simulink model "generic_20231123_1032"  (R2022b)
settings: Solver=ode45  StartTime=0.0  StopTime=50  RelTol=1e-3  EnableMultiTasking=on
model workspace (MAT data in the model file):
  A = 1
  Amplifier = -9.10007585438
  B = 1.19071237887
  K_d_yawrate = 0.231634180251
  K_dsteering = 5.24463953925
  k_speed = -0.570636497542
  k_stanley = 28.4909595466
  kd = -9.99955278144
  ki = 0.00519416981022
  kp = 9.99999979837
  path_curvature = 0
values from neighbouring files (symbols this model uses):
  brake_select = ones(length(speed), length(steering_angle))    [TwoDLook_uptable.m]
  curvature = 0.000:0.001:1    [TwoDLook_uptable.m]
  m = 1600    [MPCController1.m]    (also in MPCController2.m; MPC_Fmincon.m)
  speed = 0:0.1:100    [TwoDLook_uptable.m]
  steering_angle = -3.14/4:0.00628/4:3.14/4    [TwoDLook_uptable.m]
undefined symbols (not defined in the file or in its folder): DiscIntNeverNeededParam
libraries: CarMaker4SL x143, simulink x11, cstblocks x6, simulink_extras x4, autolibshared x1, mpcadaslib x1
(part 4 of 7)

== system generic_20231123_1032/CarMaker/VehicleControl/CreateBus VhclCtrl/Stanley steering & speed//Brake controller/Road sensor set & path planning/Road sensor set & path planning/Be'zeir path planning ==
  pathx : Inport
  path_y : Inport  Port=2
  car_v : Inport  Port=3
  Basic_obstacle avoidance : MATLAB Function  TreatAsAtomicUnit=on
  Constant : Constant  Value=10
  Constant1 : Constant  Value=1.95
  Constant2 : Constant  Value=4.2
  Demux : Demux
  Discrete-Time Integrator : DiscreteIntegrator  SampleTime=-1  ICPrevOutput=DiscIntNeverNeededParam  ICPrevScaledInput=DiscIntNeverNeededParam
  MATLAB Function : MATLAB Function  TreatAsAtomicUnit=on
  Mux : Mux  Inputs=2
  Mux1 : Mux  Inputs=2
  Read CM Dict : CarMaker4SL/Read CM Dict  xname=Sensor.Object.RadarL.Obj.T00.RefPnt.ds.x  xsync=off  xstime=Continuous
  Read CM Dict1 : CarMaker4SL/Read CM Dict  xname=Sensor.Object.RadarL.Obj.T00.RefPnt.ds.y  xsync=off  xstime=Continuous
  Read CM Dict2 : CarMaker4SL/Read CM Dict  xname=Car.Gen.tx  xsync=off  xstime=Continuous
  Read CM Dict3 : CarMaker4SL/Read CM Dict  xname=Car.Gen.ty  xsync=off  xstime=Continuous
  Read CM Dict4 : CarMaker4SL/Read CM Dict  xname=Sensor.Radar.VehSensor_6.Obj0.Width  xsync=off  xstime=Continuous
  Read CM Dict5 : CarMaker4SL/Read CM Dict  xname=Sensor.Radar.VehSensor_6.Obj0.Length  xsync=off  xstime=Continuous
  Read CM Dict6 : CarMaker4SL/Read CM Dict  xname=Car.YawRate  xsync=off  xstime=Continuous
  Reshape : Reshape  OutputDimensionality=Customize  OutputDimensions=[2,1]
  Reshape1 : Reshape  OutputDimensionality=Customize  OutputDimensions=[1,2]
  Reshape2 : Reshape  OutputDimensionality=Customize  OutputDimensions=[1,2]
  Reshape3 : Reshape  OutputDimensionality=Customize  OutputDimensions=[1,2]
  Reshape4 : Reshape
  Saturation : Saturate  UpperLimit=4  LowerLimit=-4
  Signal_smoothing : Subsystem
  Smoothing3 : Subsystem
  getInstantaneousPath Function : MATLAB Function  Commented=on  TreatAsAtomicUnit=on
  lookahead_dist : Constant  Commented=on  Value=2
  new_x_path : Outport
  new_y_path : Outport  Port=2
  wires:
  Read CM Dict1/1 -> Basic_obstacle avoidance/8(dy), MATLAB Function/4(dx)
  Read CM Dict2/1 -> Mux/1
  MATLAB Function/2(final_position) -> Reshape3/1
  Constant/1 -> MATLAB Function/5(path_length)
  Read CM Dict4/1 -> Signal_smoothing/1(Signal_In)
  Read CM Dict3/1 -> Mux/2
  Mux/1 -> Reshape/1
  Read CM Dict6/1 -> Discrete-Time Integrator/1
  Read CM Dict5/1 -> Saturation/1
  Mux1/1 -> Reshape1/1
  Read CM Dict/1 -> Basic_obstacle avoidance/7(dx), MATLAB Function/3(dy)
  Reshape/1 -> getInstantaneousPath Function/3(current_position), MATLAB Function/1(current_position)
  Discrete-Time Integrator/1 -> MATLAB Function/2(heading), getInstantaneousPath Function/4(current_heading)
  Saturation/1 -> Smoothing3/1(Signal_In)
  MATLAB Function/1(initial_position) -> Reshape2/1
  Signal_smoothing/1(smoothed_width) -> Basic_obstacle avoidance/3(obstacle_width)
  Constant1/1 -> Basic_obstacle avoidance/5(car_width)
  Smoothing3/1(Signal_Out) -> Basic_obstacle avoidance/4(obstacle_length)  "steering_signal"
  Constant2/1 -> Basic_obstacle avoidance/6(car_length)
  car_v/1 -> Basic_obstacle avoidance/9(car_v)
  path_y/1 -> Mux1/2, Basic_obstacle avoidance/11(path_y)
  pathx/1 -> Mux1/1, Basic_obstacle avoidance/10(path_x)
  lookahead_dist/1 -> getInstantaneousPath Function/2(lookahead_distance)
  Reshape2/1 -> Basic_obstacle avoidance/1(initial_position)
  Reshape3/1 -> Basic_obstacle avoidance/2(final_position)
  Demux/1 -> new_x_path/1
  Basic_obstacle avoidance/1(updated_path) -> Reshape4/1, getInstantaneousPath Function/1(generated_path)
  Demux/4 -> new_y_path/1
  Reshape4/1 -> Demux/1

== system generic_20231123_1032/CarMaker/VehicleControl/CreateBus VhclCtrl/Stanley steering & speed//Brake controller/Road sensor set & path planning/Road sensor set & path planning/Car_yaw_rate ==
  Velocity : Inport
  X-path : Inport  Port=2
  Y_path : Inport  Port=3
  " Path_expanding1" : Subsystem
  Constant : Constant  Value=20
  Gain2 : Gain  Gain=-1
  Multiport Switch : MultiPortSwitch  Inputs=2  SaturateOnIntegerOverflow=off  InputSameDT=off
  Multiport Switch1 : MultiPortSwitch  Inputs=2  SaturateOnIntegerOverflow=off  InputSameDT=off
  Product3 : Product
  Read CM Dict5 : CarMaker4SL/Read CM Dict  xname=Car.YawRate  xsync=off  xstime=Continuous
  Saturation3 : Saturate  UpperLimit=5  LowerLimit=-5
  Varying Lowpass Filter1 : cstblocks/Linear Parameter Varying/Varying Lowpass Filter  N=1
  Vehicle_yaw_rate_selcotr : Constant
  Yaw_rate_filter_slector : Constant
  calculate_path_curvature2 : MATLAB Function  TreatAsAtomicUnit=on  VariantControl=Choice
  Yaw_rate_car : Outport
  wires:
  " Path_expanding1"/1(x_path) -> calculate_path_curvature2/1(path_x)
  X-path/1 -> " Path_expanding1"/1(X-path)
  Gain2/1 -> Multiport Switch1/2, Saturation3/1
  Y_path/1 -> " Path_expanding1"/2(Y_path)
  Velocity/1 -> Product3/1
  " Path_expanding1"/2(y_path) -> calculate_path_curvature2/2(path_y)
  Product3/1 -> Gain2/1
  calculate_path_curvature2/1(path_curvature) -> Product3/2
  Saturation3/1 -> Varying Lowpass Filter1/1
  Constant/1 -> Varying Lowpass Filter1/2
  Yaw_rate_filter_slector/1 -> Multiport Switch1/1
  Varying Lowpass Filter1/1 -> Multiport Switch1/3  "Yaw_rate_car"
  Vehicle_yaw_rate_selcotr/1 -> Multiport Switch/1
  Multiport Switch1/1 -> Multiport Switch/2
  Read CM Dict5/1 -> Multiport Switch/3
  Multiport Switch/1 -> Yaw_rate_car/1  "Yaw_rate_car"

== system generic_20231123_1032/CarMaker/VehicleControl/CreateBus VhclCtrl/Stanley steering & speed//Brake controller/Road sensor set & path planning/Road sensor set & path planning/Cross_track_error_calcuation ==
  x_path : Inport
  y_path : Inport  Port=2
  Constant : Constant  Value=25
  Cross_track_error_calcuation : MATLAB Function  TreatAsAtomicUnit=on
  Delay : Delay  DelayLength=1  InitialCondition=0.1
  Delay1 : Delay  DelayLength=1  InitialCondition=0.1
  Gain1 : Gain  Gain=-1
  Read CM Dict12 : CarMaker4SL/Read CM Dict  xname=Car.Gen.ty  xsync=off  xstime=Continuous
  Read CM Dict8 : CarMaker4SL/Read CM Dict  xname=Car.Gen.tx  xsync=off  xstime=Continuous
  Saturation1 : Saturate  UpperLimit=7  LowerLimit=-7
  Varying Lowpass Filter2 : cstblocks/Linear Parameter Varying/Varying Lowpass Filter  N=1
  cte : Outport
  denominator : Outport  Port=2
  wires:
  Read CM Dict12/1 -> Cross_track_error_calcuation/2(y_vehicle)
  x_path/1 -> Cross_track_error_calcuation/5(x2), Delay1/1
  Saturation1/1 -> Varying Lowpass Filter2/1
  Delay/1 -> Cross_track_error_calcuation/4(y_point)
  Cross_track_error_calcuation/2(denominator) -> denominator/1
  y_path/1 -> Cross_track_error_calcuation/6(y2), Delay/1
  Delay1/1 -> Cross_track_error_calcuation/3(x_point)
  Read CM Dict8/1 -> Cross_track_error_calcuation/1(x_vehicle)
  Cross_track_error_calcuation/1(cte) -> Gain1/1
  Gain1/1 -> Saturation1/1
  Constant/1 -> Varying Lowpass Filter2/2
  Varying Lowpass Filter2/1 -> cte/1

== system generic_20231123_1032/CarMaker/VehicleControl/CreateBus VhclCtrl/Stanley steering & speed//Brake controller/Road sensor set & path planning/Road sensor set & path planning/Dijkestra path planning ==
  path_y : Inport
  car_v : Inport  Port=2
  pathx : Inport  Port=3
  Basic_obstacle avoidance : MATLAB Function  TreatAsAtomicUnit=on
  Demux : Demux  Commented=on
  Discrete-Time Integrator : DiscreteIntegrator  SampleTime=-1  ICPrevOutput=DiscIntNeverNeededParam  ICPrevScaledInput=DiscIntNeverNeededParam
  Mux : Mux  Inputs=2
  Mux1 : Mux  Inputs=2
  Read CM Dict : CarMaker4SL/Read CM Dict  xname=Sensor.Object.RadarL.Obj.T00.RefPnt.ds.x  xsync=off  xstime=Continuous
  Read CM Dict1 : CarMaker4SL/Read CM Dict  xname=Sensor.Object.RadarL.Obj.T00.RefPnt.ds.y  xsync=off  xstime=Continuous
  Read CM Dict2 : CarMaker4SL/Read CM Dict  xname=Car.Gen.tx  xsync=off  xstime=Continuous
  Read CM Dict3 : CarMaker4SL/Read CM Dict  xname=Car.Gen.ty  xsync=off  xstime=Continuous
  Read CM Dict4 : CarMaker4SL/Read CM Dict  xname=Sensor.Radar.VehSensor_6.Obj0.Width  xsync=off  xstime=Continuous
  Read CM Dict5 : CarMaker4SL/Read CM Dict  xname=Sensor.Radar.VehSensor_6.Obj0.Length  xsync=off  xstime=Continuous
  Read CM Dict6 : CarMaker4SL/Read CM Dict  xname=Car.YawRate  xsync=off  xstime=Continuous
  Reshape : Reshape  OutputDimensionality=Customize  OutputDimensions=[2,1]
  Reshape1 : Reshape  OutputDimensionality=Customize  OutputDimensions=[1,2]
  Reshape4 : Reshape  Commented=on
  Saturation : Saturate  UpperLimit=4  LowerLimit=-4
  Signal_smoothing : Subsystem
  Smoothing3 : Subsystem
  getInstantaneousPath Function : MATLAB Function  Commented=on  TreatAsAtomicUnit=on
  lookahead_dist : Constant  Commented=on  Value=2
  new_x_path : Outport
  new_y_path : Outport  Port=2
  wires:
  Read CM Dict/1 -> Basic_obstacle avoidance/3(dx)
  Read CM Dict1/1 -> Basic_obstacle avoidance/4(dy)
  Read CM Dict2/1 -> Mux/1, Basic_obstacle avoidance/1(Car_x)
  Read CM Dict4/1 -> Signal_smoothing/1(Signal_In)
  Read CM Dict3/1 -> Mux/2, Basic_obstacle avoidance/2(Car_y)
  Mux/1 -> Reshape/1
  Read CM Dict6/1 -> Discrete-Time Integrator/1
  Read CM Dict5/1 -> Saturation/1
  Mux1/1 -> Reshape1/1
  Reshape/1 -> getInstantaneousPath Function/3(current_position)
  Discrete-Time Integrator/1 -> getInstantaneousPath Function/4(current_heading)
  Saturation/1 -> Smoothing3/1(Signal_In)
  Signal_smoothing/1(smoothed_width) -> Basic_obstacle avoidance/6(object_width)
  Smoothing3/1(Signal_Out) -> Basic_obstacle avoidance/5(object_length)  "steering_signal"
  car_v/1 -> Basic_obstacle avoidance/7(car_v)
  path_y/1 -> Mux1/2, Basic_obstacle avoidance/9(path_y)
  pathx/1 -> Mux1/1, Basic_obstacle avoidance/8(path_x)
  lookahead_dist/1 -> getInstantaneousPath Function/2(lookahead_distance)
  Demux/1 -> new_x_path/1
  Basic_obstacle avoidance/1(updated_path) -> Reshape4/1, getInstantaneousPath Function/1(generated_path)
  Demux/4 -> new_y_path/1
  Reshape4/1 -> Demux/1

== system generic_20231123_1032/CarMaker/VehicleControl/CreateBus VhclCtrl/Stanley steering & speed//Brake controller/Road sensor set & path planning/Road sensor set & path planning/Path_curvature ==
  X-path : Inport
  Y_path : Inport  Port=2
  " Path_expanding" : Subsystem
  Constant : Constant  Value=25
  Multiport Switch : MultiPortSwitch  Inputs=2  SaturateOnIntegerOverflow=off  InputSameDT=off
  Multiport Switch1 : MultiPortSwitch  Inputs=2  SaturateOnIntegerOverflow=off  InputSameDT=off
  Read CM Dict6 : CarMaker4SL/Read CM Dict  xname=Sensor.Road.VehSensor_0.Path.CurveXY  xsync=off  xstime=Continuous
  Saturation2 : Saturate  UpperLimit=1  LowerLimit=-1
  Scope : Scope
  Varying Lowpass Filter : cstblocks/Linear Parameter Varying/Varying Lowpass Filter  N=1
  calculate_path_curvature1 : MATLAB Function  TreatAsAtomicUnit=on  VariantControl=Choice
  inverting : Gain  Gain=-1
  path_curv_selector : Constant
  path_curv_selector1 : Constant
  Path_curvature : Outport
  smoothed_path_curvature : Outport  Port=2
  wires:
  inverting/1 -> Multiport Switch1/2, Saturation2/1
  X-path/1 -> " Path_expanding"/1(X-path)
  Y_path/1 -> " Path_expanding"/2(Y_path)
  " Path_expanding"/1(x_path) -> calculate_path_curvature1/1(path_x)
  calculate_path_curvature1/1(path_curvature) -> inverting/1
  Read CM Dict6/1 -> Multiport Switch/3
  " Path_expanding"/2(y_path) -> calculate_path_curvature1/2(path_y)
  Saturation2/1 -> Varying Lowpass Filter/1
  Varying Lowpass Filter/1 -> Scope/1, smoothed_path_curvature/1, Multiport Switch1/3  "Path_curvature"
  Constant/1 -> Varying Lowpass Filter/2
  path_curv_selector1/1 -> Multiport Switch1/1
  path_curv_selector/1 -> Multiport Switch/1
  Multiport Switch1/1 -> Multiport Switch/2
  Multiport Switch/1 -> Path_curvature/1  "Path_curvature"

== system generic_20231123_1032/CarMaker/VehicleControl/CreateBus VhclCtrl/Stanley steering & speed//Brake controller/Road sensor set & path planning/Road sensor set & path planning/Spline_path_planning ==
  Velocity : Inport
  pathx : Inport  Port=2
  path_y : Inport  Port=3
  Demux : Demux  Outputs=2
  Discrete-Time Integrator : DiscreteIntegrator  SampleTime=-1  ICPrevOutput=DiscIntNeverNeededParam  ICPrevScaledInput=DiscIntNeverNeededParam
  Mux : Mux  Inputs=2
  Mux1 : Mux  Inputs=2
  Read CM Dict : CarMaker4SL/Read CM Dict  xname=Sensor.Object.RadarL.Obj.T00.RefPnt.ds.x  xsync=off  xstime=Continuous
  Read CM Dict1 : CarMaker4SL/Read CM Dict  xname=Sensor.Object.RadarL.Obj.T00.RefPnt.ds.y  xsync=off  xstime=Continuous
  Read CM Dict2 : CarMaker4SL/Read CM Dict  xname=Car.Gen.tx  xsync=off  xstime=Continuous
  Read CM Dict3 : CarMaker4SL/Read CM Dict  xname=Car.Gen.ty  xsync=off  xstime=Continuous
  Read CM Dict4 : CarMaker4SL/Read CM Dict  xname=Sensor.Radar.VehSensor_6.Obj0.Width  xsync=off  xstime=Continuous
  Read CM Dict5 : CarMaker4SL/Read CM Dict  xname=Sensor.Radar.VehSensor_6.Obj0.Length  xsync=off  xstime=Continuous
  Read CM Dict6 : CarMaker4SL/Read CM Dict  xname=Car.YawRate  xsync=off  xstime=Continuous
  Reshape : Reshape  OutputDimensionality=Customize  OutputDimensions=[1,2]
  Reshape1 : Reshape  OutputDimensionality=Customize  OutputDimensions=[1,2]
  Saturation : Saturate  UpperLimit=4  LowerLimit=-4
  Signal_smoothing : Subsystem
  Smoothing3 : Subsystem
  Spline_bsed_obstacle avoidance : MATLAB Function  TreatAsAtomicUnit=on
  getInstantaneousPath Function : MATLAB Function  TreatAsAtomicUnit=on
  lookahead_dist : Constant  Value=2
  new_x_path : Outport
  new_y_path : Outport  Port=2
  wires:
  Signal_smoothing/1(smoothed_width) -> Spline_bsed_obstacle avoidance/5(object_width)
  Read CM Dict4/1 -> Signal_smoothing/1(Signal_In)
  Demux/1 -> new_x_path/1
  Demux/2 -> new_y_path/1
  Spline_bsed_obstacle avoidance/1(updated_path) -> getInstantaneousPath Function/1(generated_path)  "generated_path"
  Smoothing3/1(Signal_Out) -> Spline_bsed_obstacle avoidance/6(object_length)  "steering_signal"
  Read CM Dict1/1 -> Spline_bsed_obstacle avoidance/4(dy)
  Read CM Dict/1 -> Spline_bsed_obstacle avoidance/3(dx)
  Saturation/1 -> Smoothing3/1(Signal_In)
  Velocity/1 -> Spline_bsed_obstacle avoidance/7(car_v)
  Read CM Dict5/1 -> Saturation/1
  Read CM Dict3/1 -> Mux/2, Spline_bsed_obstacle avoidance/2(Car_y)  "car_y"
  Read CM Dict2/1 -> Mux/1, Spline_bsed_obstacle avoidance/1(Car_x)  "car_x"
  Mux/1 -> Reshape/1
  Reshape/1 -> getInstantaneousPath Function/3(current_position)
  lookahead_dist/1 -> getInstantaneousPath Function/2(lookahead_distance)
  Read CM Dict6/1 -> Discrete-Time Integrator/1
  Discrete-Time Integrator/1 -> getInstantaneousPath Function/4(current_heading)
  Mux1/1 -> Reshape1/1
  pathx/1 -> Spline_bsed_obstacle avoidance/8(pathx), Mux1/1
  path_y/1 -> Spline_bsed_obstacle avoidance/9(path_y), Mux1/2
  getInstantaneousPath Function/1(instantaneous_points) -> Demux/1

== system generic_20231123_1032/CarMaker/VehicleControl/CreateBus VhclCtrl/Stanley steering & speed//Brake controller/Road sensor set & path planning/Road sensor set & path planning/path_planning ==
  <tx> : Inport
  <ty> : Inport  Port=2
  Velocity : Inport  Port=3
  Basic_obstacle avoidance : MATLAB Function  TreatAsAtomicUnit=on
  Demux : Demux  Outputs=2
  Floor : Rounding  Operator=ceil
  Read CM Dict : CarMaker4SL/Read CM Dict  xname=Sensor.Object.RadarL.Obj.T00.RefPnt.ds.x  xsync=off  xstime=Continuous
  Read CM Dict1 : CarMaker4SL/Read CM Dict  xname=Sensor.Object.RadarL.Obj.T00.RefPnt.ds.y  xsync=off  xstime=Continuous
  Read CM Dict2 : CarMaker4SL/Read CM Dict  xname=Car.Gen.tx  xsync=off  xstime=Continuous
  Read CM Dict3 : CarMaker4SL/Read CM Dict  xname=Car.Gen.ty  xsync=off  xstime=Continuous
  Read CM Dict4 : CarMaker4SL/Read CM Dict  xname=Sensor.Radar.VehSensor_6.Obj0.Width  xsync=off  xstime=Continuous
  Read CM Dict5 : CarMaker4SL/Read CM Dict  xname=Sensor.Radar.VehSensor_6.Obj0.Length  xsync=off  xstime=Continuous
  Saturation : Saturate  UpperLimit=4  LowerLimit=-4
  Signal_smoothing : Subsystem
  Smoothing3 : Subsystem
  To Workspace1 : ToWorkspace  Commented=on  VariableName=CarY  SampleTime=-1
      settings: Save2DSignal=2-D array (concatenate along first dimension)
  To Workspace3 : ToWorkspace  Commented=on  VariableName=CarX  SampleTime=-1
      settings: Save2DSignal=2-D array (concatenate along first dimension)
  new_x_path : Outport
  new_y_path : Outport  Port=2
  wires:
  Read CM Dict2/1 -> To Workspace3/1, Basic_obstacle avoidance/1(Car_x)
  Read CM Dict3/1 -> To Workspace1/1, Basic_obstacle avoidance/2(Car_y)
  Read CM Dict5/1 -> Saturation/1
  Velocity/1 -> Basic_obstacle avoidance/9(car_v), Floor/1
  Saturation/1 -> Smoothing3/1(Signal_In)
  Read CM Dict/1 -> Basic_obstacle avoidance/3(dx)
  Read CM Dict1/1 -> Basic_obstacle avoidance/4(dy)
  Smoothing3/1(Signal_Out) -> Basic_obstacle avoidance/6(object_length)  "steering_signal"
  <tx>/1 -> Basic_obstacle avoidance/7(path_x)
  <ty>/1 -> Basic_obstacle avoidance/8(path_y)
  Floor/1 -> Basic_obstacle avoidance/10(car_v_ceil)
  Basic_obstacle avoidance/1(updated_path) -> Demux/1
  Demux/2 -> new_y_path/1
  Demux/1 -> new_x_path/1
  Read CM Dict4/1 -> Signal_smoothing/1(Signal_In)
  Signal_smoothing/1(smoothed_width) -> Basic_obstacle avoidance/5(object_width)

== system generic_20231123_1032/CarMaker/VehicleControl/CreateBus VhclCtrl/Stanley steering & speed//Brake controller/Stanley controller with path_planning/Stanley controller with path_planning/Subsystem3 ==
  X-path : Inport
  Y_path : Inport  Port=2
  Delay37 : Delay  DelayLength=1
  Delay4 : Delay  DelayLength=1
  Mux1 : Mux  Inputs=2
  Mux2 : Mux  Inputs=2
  Reshape1 : Reshape  OutputDimensionality=Customize  OutputDimensions=[1,2]
  Reshape2 : Reshape  OutputDimensionality=Customize  OutputDimensions=[1,2]
  x_path : Outport
  y_path : Outport  Port=2
  wires:
  X-path/1 -> Delay37/1, Mux2/1
  Y_path/1 -> Delay4/1, Mux1/1
  Delay37/1 -> Mux2/2
  Mux1/1 -> Reshape1/1
  Reshape1/1 -> y_path/1
  Delay4/1 -> Mux1/2
  Reshape2/1 -> x_path/1
  Mux2/1 -> Reshape2/1

== system generic_20231123_1032/CarMaker/VehicleControl/CreateBus VhclCtrl/Stanley steering & speed//Brake controller/Stanley controller with path_planning/Stanley controller with path_planning/X_Global_Pos_m ==
  In1 : Inport
  Pos_X : Outport  VectorParamsAs1DForOutWhenUnconnected=off
  wires:
  In1/1 -> Pos_X/1

== system generic_20231123_1032/CarMaker/VehicleControl/CreateBus VhclCtrl/Stanley steering & speed//Brake controller/Stanley controller with path_planning/Stanley controller with path_planning/Y_Global_Pos_m ==
  In1 : Inport
  Pos_Y : Outport  VectorParamsAs1DForOutWhenUnconnected=off
  wires:
  In1/1 -> Pos_Y/1

== system generic_20231123_1032/CarMaker/VehicleControl/CreateBus VhclCtrl/Stanley steering & speed//Brake controller/Stanley controller with path_planning/Stanley controller with path_planning/Yaw_angle_rad ==
  In1 : Inport
  Yaw_Angle : Outport  VectorParamsAs1DForOutWhenUnconnected=off
  wires:
  In1/1 -> Yaw_Angle/1

== system generic_20231123_1032/CarMaker/VehicleControl/CreateBus VhclCtrl/Stanley steering & speed//Brake controller/Stanley_controller_vfin/Stanley_controller_vfin/Stanley_standfort controller ==
  note: Vehicle_paramters
  note: Parameters
  note: K_dsteering = 10;
  note: Amplifier = -5.94
  note: K_d_yawrate =0.4
  note: Vehicle overall mass [kg] 	: 	1600.00
      |
      |  Vehicle overall center of gravity x / y / z [m] 	: 	2.596	0.000	0.562
      |
      |  Vehicle overall inertia tensor [kgm²] 	: 	696.215	0.000	-8.863
      |  	 									0.000	2707.206	0.000
      |  	 									-8.863	0.000	2986.624
  note: Distance CoG to front axle / rear axle [m] : 1.488 -1.487
  note: k_stanly = 13.6;
  Velocity : Inport
  Curvature : Inport  Port=2
  Vehicle_yaw_rate : Inport  Port=3
  Path.DevDist : Inport  Port=4
  Add : Sum  Inputs=+++
  Add1 : Sum
  Crosstrack_steering : Subsystem
  Deviation_angle_calc : Subsystem
  Scope : Scope  NumInputPorts=2
  Steady_state_yaw : Subsystem  Commented=on
  Steering_correction_facotr : Subsystem
  Yaw_rate_diff : Subsystem
  Steering angle : Outport
  dev_angle : Outport  Port=2
  wires:
  Velocity/1 -> Crosstrack_steering/1(speed), Deviation_angle_calc/1(Velocity), Yaw_rate_diff/1(Velocity)
  Crosstrack_steering/1(Cross_track_steering) -> Add/1  "Crosstrack_steering"
  Add/1 -> Add1/1
  Add1/1 -> Steering angle/1, Steering_correction_facotr/1(Steering_i+1), Steering_correction_facotr/2(Steering_i)  "Steering angle"
  Deviation_angle_calc/1(Dev_angle) -> dev_angle/1, Add/3
  Steering_correction_facotr/1(Factor_of_correction) -> Add1/2
  Yaw_rate_diff/1(Yaw_rate_factor) -> Add/2
  Vehicle_yaw_rate/1 -> Yaw_rate_diff/3(Car_yaw_rate), Deviation_angle_calc/3(Car.YawRate), Scope/2
  Path.DevDist/1 -> Crosstrack_steering/2(Path.DevDist)
  Curvature/1 -> Scope/1, Deviation_angle_calc/2(Curvature), Yaw_rate_diff/2(Curvature)

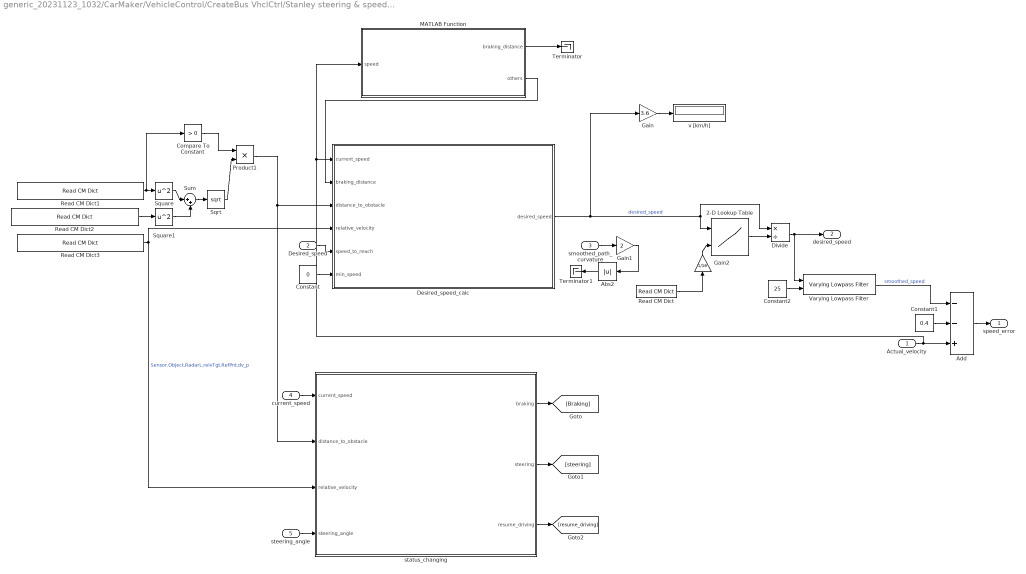
== system generic_20231123_1032/CarMaker/VehicleControl/CreateBus VhclCtrl/Stanley steering & speed//Brake controller/Stanley_controller_with_thottle_and_brake_commands/MPCLongitudianl_contorl/Speed_regulator ==
  Actual_velocity : Inport
  Desired_speed : Inport  Port=2
  smoothed_path_curvature : Inport  Port=3
  current_speed : Inport  Port=4
  steering_angle : Inport  Port=5
  2-D Lookup Table : Lookup_n-D  BreakpointsForDimension1=speed  BreakpointsForDimension2=steering_angle  Table=brake_select  InternalRulePriority=Speed  RndMeth=Simplest
      settings: InputPortMap=u0,u1
  Abs2 : Abs  SaturateOnIntegerOverflow=off
  Add : Sum  Inputs=--+
  Compare To Constant : simulink/Logic and Bit Operations/Compare To Constant  relop=>  const=0  OutDataTypeStr=boolean
  Constant : Constant  Value=0
  Constant1 : Constant  Value=0.4
  Constant2 : Constant  Value=25
  Desired_speed_calc : MATLAB Function  TreatAsAtomicUnit=on
  Divide : Product  Inputs=*/
  Gain : Gain  Gain=3.6
  Gain1 : Gain  Gain=2
  Gain2 : Gain  Gain=1/16
  MATLAB Function : MATLAB Function  TreatAsAtomicUnit=on
  Product1 : Product
  Read CM Dict : CarMaker4SL/Read CM Dict  xname=Steer.WhlAng  xsync=off  xstime=Continuous
  Read CM Dict1 : CarMaker4SL/Read CM Dict  xname=Sensor.Object.RadarL.Obj.T01.RefPnt.ds.x  xsync=off  xstime=Continuous
  Read CM Dict2 : CarMaker4SL/Read CM Dict  xname=Sensor.Object.RadarL.Obj.T01.RefPnt.ds.y  xsync=off  xstime=Continuous
  Read CM Dict3 : CarMaker4SL/Read CM Dict  xname=Sensor.Object.RadarL.relvTgt.RefPnt.dv_p  xsync=off  xstime=Continuous
  Sqrt : Sqrt
  Square : Math  Operator=square
  Square1 : Math  Operator=square
  Sum : Sum  Inputs=|++
  Terminator : Terminator
  Terminator1 : Terminator
  Varying Lowpass Filter : cstblocks/Linear Parameter Varying/Varying Lowpass Filter  N=1
  status_changing : MATLAB Function  TreatAsAtomicUnit=on
  v [km/h] : Display
  speed_error : Outport
  desired_speed : Outport  Port=2
  wires:
  Gain1/1 -> Abs2/1
  Constant/1 -> Desired_speed_calc/6(min_speed)
  Sqrt/1 -> Product1/2
  Desired_speed/1 -> Desired_speed_calc/5(speed_to_reach)
  Read CM Dict3/1 -> status_changing/3(relative_velocity), Desired_speed_calc/4(relative_velocity)  "Sensor.Object.RadarL.relvTgt.RefPnt.dv_p"
  Constant1/1 -> Add/2
  Product1/1 -> status_changing/2(distance_to_obstacle), Desired_speed_calc/3(distance_to_obstacle)
  Desired_speed_calc/1(desired_speed) -> Gain/1, Divide/1, 2-D Lookup Table/1  "desired_speed"
  Read CM Dict2/1 -> Square1/1
  steering_angle/1 -> status_changing/4(steering_angle)
  Square1/1 -> Sum/2
  Gain/1 -> v [km/h]/1
  2-D Lookup Table/1 -> Divide/2
  status_changing/3(resume_driving) -> [resume_driving]
  Sum/1 -> Sqrt/1
  Square/1 -> Sum/1
  Add/1 -> speed_error/1
  smoothed_path_curvature/1 -> Gain1/1
  Compare To Constant/1 -> Product1/1
  Read CM Dict1/1 -> Compare To Constant/1, Square/1
  status_changing/2(steering) -> [steering]
  status_changing/1(braking) -> [Braking]
  current_speed/1 -> status_changing/1(current_speed)
  Constant2/1 -> Varying Lowpass Filter/2
  Divide/1 -> desired_speed/1, Varying Lowpass Filter/1
  Varying Lowpass Filter/1 -> Add/1  "smoothed_speed"
  Actual_velocity/1 -> MATLAB Function/1(speed), Desired_speed_calc/1(current_speed), Add/3
  MATLAB Function/2(others) -> Desired_speed_calc/2(braking_distance)
  MATLAB Function/1(braking_distance) -> Terminator/1
  Abs2/1 -> Terminator1/1
  Read CM Dict/1 -> Gain2/1
  Gain2/1 -> 2-D Lookup Table/2

== system generic_20231123_1032/CarMaker/VehicleControl/CreateBus VhclCtrl/Stanley steering & speed//Brake controller/Stanley_controller_with_thottle_and_brake_commands/Stanley steering + PID speed controller/Smoothing ==
  Signal_In : Inport
  Add : Sum  Inputs=++++
  Delay : Delay  InitialCondition=0.1
  Delay1 : Delay  DelayLength=4  InitialCondition=0.1
  Delay2 : Delay  DelayLength=5  InitialCondition=0.1
  Gain : Gain  Gain=0.35
  Gain1 : Gain  Gain=0.25
  Gain2 : Gain  Gain=0.25
  Gain3 : Gain  Gain=0.15
  Signal_Out : Outport  VectorParamsAs1DForOutWhenUnconnected=off
  wires:
  Gain1/1 -> Add/2
  Signal_In/1 -> Gain/1
  Delay/1 -> Gain1/1
  Gain/1 -> Add/1
  Delay1/1 -> Gain2/1
  Add/1 -> Delay2/1, Delay1/1, Delay/1, Signal_Out/1
  Gain2/1 -> Add/3
  Delay2/1 -> Gain3/1
  Gain3/1 -> Add/4

== system generic_20231123_1032/CarMaker/VehicleControl/CreateBus VhclCtrl/Stanley steering & speed//Brake controller/Stanley_controller_with_thottle_and_brake_commands/Stanley steering + PID speed controller/Speed_controller ==
  path : Inport
  speed_act : Inport  Port=2
  velocity_x : Inport  Port=3
  velocity_y : Inport  Port=4
  desired_speed : Inport  Port=5
  steering : Inport  Port=6
  Brake Saturation : Saturate  UpperLimit=1  LowerLimit=0
  Constant1 : Constant  Value=kd
  Constant2 : Constant  Value=ki
  Constant3 : Constant  Value=kp
  Path_curvature : Constant  Value=path_curvature
  Scaling factor : Gain  Gain=1/1000
  Scalling factor : Gain  Gain=1/1000
  Throttle Saturation : Saturate  UpperLimit=1  LowerLimit=-1
  advancedPID_speed_and_brake_control : MATLAB Function  TreatAsAtomicUnit=on
  calculate_path_curvature : MATLAB Function  TreatAsAtomicUnit=on
  Throttle : Outport
  Brake_command : Outport  Port=2
  path_curvature : Outport  Port=3
  min_safe_speed : Outport  Port=4
  wires:
  advancedPID_speed_and_brake_control/1(throttle) -> Scaling factor/1  "throttle"
  path/1 -> calculate_path_curvature/1(path)
  speed_act/1 -> advancedPID_speed_and_brake_control/3(speed_act)
  calculate_path_curvature/2(min_safe_speed) -> min_safe_speed/1, advancedPID_speed_and_brake_control/2(min_s_speed)  "min_s_speed"
  velocity_y/1 -> calculate_path_curvature/2(velocity_y)
  velocity_x/1 -> calculate_path_curvature/3(velocity_x)
  steering/1 -> calculate_path_curvature/4(steering_angel)
  calculate_path_curvature/1(path_curvature) -> path_curvature/1
  Constant3/1 -> advancedPID_speed_and_brake_control/7(Kp_speed)
  Path_curvature/1 -> advancedPID_speed_and_brake_control/1(path_curv)
  desired_speed/1 -> advancedPID_speed_and_brake_control/4(desired_speed)
  Constant2/1 -> advancedPID_speed_and_brake_control/6(Ki_speed)
  Constant1/1 -> advancedPID_speed_and_brake_control/5(Kd_speed)
  advancedPID_speed_and_brake_control/2(brake_cmd) -> Scalling factor/1  "Brake cmd"
  Scaling factor/1 -> Throttle Saturation/1
  Throttle Saturation/1 -> Throttle/1  "Throttle_command"
  Scalling factor/1 -> Brake Saturation/1
  Brake Saturation/1 -> Brake_command/1  "Brake_command"

== system generic_20231123_1032/CarMaker/VehicleControl/CreateBus VhclCtrl/Stanley steering & speed//Brake controller/Stanley_controller_with_thottle_and_brake_commands/Stanley steering + PID speed controller/Subsystem1 ==
  desired_speed : Inport
  curvature : Inport  Port=2
  min_safe_speed : Inport  Port=3
  2-D Lookup Table : Lookup_n-D  BreakpointsForDimension1=speed  BreakpointsForDimension2=curvature  Table=brake_select  InternalRulePriority=Speed  RndMeth=Simplest
      settings: InputPortMap=u0,u1
  Divide : Product  Inputs=*/
  MATLAB Function : MATLAB Function  Commented=on  TreatAsAtomicUnit=on
  Read CM Dict : CarMaker4SL/Read CM Dict  xname=Sensor.Road.VehSensor_0.Path.CurveXY  xsync=off  xstime=Continuous
  Scope2 : Scope
  Target_speed : Outport
  curv : Outport  Port=2
  speed : Outport  Port=3
  wires:
  Divide/1 -> speed/1, Target_speed/1, Scope2/1
  2-D Lookup Table/1 -> Divide/2
  desired_speed/1 -> 2-D Lookup Table/1, Divide/1
  min_safe_speed/1 -> MATLAB Function/2(min_safe_speed)
  curvature/1 -> MATLAB Function/1(u)
  Read CM Dict/1 -> curv/1, 2-D Lookup Table/2

== system generic_20231123_1032/CarMaker/VehicleControl/CreateBus VhclCtrl/Stanley steering & speed//Brake controller/Road sensor set & path planning/Road sensor set & path planning/A* star path planning/Signal_smoothing ==
  Signal_In : Inport
  Smoothing1 : Subsystem
  Smoothing2 : Subsystem
  Smoothing4 : Subsystem
  smoothed_width : Outport
  wires:
  Signal_In/1 -> Smoothing1/1(Signal_In)
  Smoothing1/1(Signal_Out) -> Smoothing2/1(Signal_In)  "steering_signal"
  Smoothing2/1(Signal_Out) -> Smoothing4/1(Signal_In)  "steering_signal"
  Smoothing4/1(Signal_Out) -> smoothed_width/1  "smoothed_width"

== system generic_20231123_1032/CarMaker/VehicleControl/CreateBus VhclCtrl/Stanley steering & speed//Brake controller/Road sensor set & path planning/Road sensor set & path planning/A* star path planning/Smoothing3 ==
  Signal_In : Inport
  Add : Sum  Inputs=++++
  Delay : Delay  InitialCondition=0.1
  Delay1 : Delay  DelayLength=4  InitialCondition=0.1
  Delay2 : Delay  DelayLength=5  InitialCondition=0.1
  Gain : Gain  Gain=0.35
  Gain1 : Gain  Gain=0.25
  Gain2 : Gain  Gain=0.25
  Gain3 : Gain  Gain=0.15
  Signal_Out : Outport  VectorParamsAs1DForOutWhenUnconnected=off
  wires:
  Gain3/1 -> Add/4
  Delay2/1 -> Gain3/1
  Gain2/1 -> Add/3
  Add/1 -> Signal_Out/1, Delay/1, Delay1/1, Delay2/1
  Delay1/1 -> Gain2/1
  Gain/1 -> Add/1
  Delay/1 -> Gain1/1
  Signal_In/1 -> Gain/1
  Gain1/1 -> Add/2

== system generic_20231123_1032/CarMaker/VehicleControl/CreateBus VhclCtrl/Stanley steering & speed//Brake controller/Road sensor set & path planning/Road sensor set & path planning/Be'zeir path planning/Signal_smoothing ==
  Signal_In : Inport
  Smoothing1 : Subsystem
  Smoothing2 : Subsystem
  Smoothing4 : Subsystem
  smoothed_width : Outport
  wires:
  Smoothing4/1(Signal_Out) -> smoothed_width/1  "smoothed_width"
  Smoothing2/1(Signal_Out) -> Smoothing4/1(Signal_In)  "steering_signal"
  Smoothing1/1(Signal_Out) -> Smoothing2/1(Signal_In)  "steering_signal"
  Signal_In/1 -> Smoothing1/1(Signal_In)

== system generic_20231123_1032/CarMaker/VehicleControl/CreateBus VhclCtrl/Stanley steering & speed//Brake controller/Road sensor set & path planning/Road sensor set & path planning/Be'zeir path planning/Smoothing3 ==
  Signal_In : Inport
  Add : Sum  Inputs=++++
  Delay : Delay  InitialCondition=0.1
  Delay1 : Delay  DelayLength=4  InitialCondition=0.1
  Delay2 : Delay  DelayLength=5  InitialCondition=0.1
  Gain : Gain  Gain=0.35
  Gain1 : Gain  Gain=0.25
  Gain2 : Gain  Gain=0.25
  Gain3 : Gain  Gain=0.15
  Signal_Out : Outport  VectorParamsAs1DForOutWhenUnconnected=off
  wires:
  Gain1/1 -> Add/2
  Signal_In/1 -> Gain/1
  Delay/1 -> Gain1/1
  Gain/1 -> Add/1
  Delay1/1 -> Gain2/1
  Add/1 -> Delay2/1, Delay1/1, Delay/1, Signal_Out/1
  Gain2/1 -> Add/3
  Delay2/1 -> Gain3/1
  Gain3/1 -> Add/4

== system generic_20231123_1032/CarMaker/VehicleControl/CreateBus VhclCtrl/Stanley steering & speed//Brake controller/Road sensor set & path planning/Road sensor set & path planning/Car_yaw_rate/ Path_expanding1 ==
  X-path : Inport
  Y_path : Inport  Port=2
  Delay10 : Delay  DelayLength=6
  Delay11 : Delay  DelayLength=8
  Delay37 : Delay
  Delay38 : Delay  DelayLength=4
  Delay4 : Delay
  Delay5 : Delay  DelayLength=6
  Delay6 : Delay  DelayLength=8
  Delay9 : Delay  DelayLength=4
  Mux1 : Mux  Inputs=5
  Mux2 : Mux  Inputs=5
  Reshape1 : Reshape  OutputDimensionality=Customize  OutputDimensions=[1,5]
  Reshape2 : Reshape  OutputDimensionality=Customize  OutputDimensions=[1,5]
  x_path : Outport
  y_path : Outport  Port=2
  wires:
  Mux2/1 -> Reshape2/1
  Reshape2/1 -> x_path/1
  Delay11/1 -> Mux1/5
  Delay10/1 -> Mux1/4
  Delay9/1 -> Mux1/3
  Delay4/1 -> Mux1/2
  Reshape1/1 -> y_path/1
  Mux1/1 -> Reshape1/1
  Delay38/1 -> Mux2/3
  Delay6/1 -> Mux2/5
  Delay37/1 -> Mux2/2
  Delay5/1 -> Mux2/4
  Y_path/1 -> Delay11/1, Delay10/1, Delay9/1, Delay4/1, Mux1/1
  X-path/1 -> Delay6/1, Delay5/1, Delay37/1, Delay38/1, Mux2/1

== system generic_20231123_1032/CarMaker/VehicleControl/CreateBus VhclCtrl/Stanley steering & speed//Brake controller/Road sensor set & path planning/Road sensor set & path planning/Dijkestra path planning/Signal_smoothing ==
  Signal_In : Inport
  Smoothing1 : Subsystem
  Smoothing2 : Subsystem
  Smoothing4 : Subsystem
  smoothed_width : Outport
  wires:
  Smoothing4/1(Signal_Out) -> smoothed_width/1  "smoothed_width"
  Smoothing2/1(Signal_Out) -> Smoothing4/1(Signal_In)  "steering_signal"
  Smoothing1/1(Signal_Out) -> Smoothing2/1(Signal_In)  "steering_signal"
  Signal_In/1 -> Smoothing1/1(Signal_In)

== system generic_20231123_1032/CarMaker/VehicleControl/CreateBus VhclCtrl/Stanley steering & speed//Brake controller/Road sensor set & path planning/Road sensor set & path planning/Dijkestra path planning/Smoothing3 ==
  Signal_In : Inport
  Add : Sum  Inputs=++++
  Delay : Delay  InitialCondition=0.1
  Delay1 : Delay  DelayLength=4  InitialCondition=0.1
  Delay2 : Delay  DelayLength=5  InitialCondition=0.1
  Gain : Gain  Gain=0.35
  Gain1 : Gain  Gain=0.25
  Gain2 : Gain  Gain=0.25
  Gain3 : Gain  Gain=0.15
  Signal_Out : Outport  VectorParamsAs1DForOutWhenUnconnected=off
  wires:
  Gain1/1 -> Add/2
  Signal_In/1 -> Gain/1
  Delay/1 -> Gain1/1
  Gain/1 -> Add/1
  Delay1/1 -> Gain2/1
  Add/1 -> Delay2/1, Delay1/1, Delay/1, Signal_Out/1
  Gain2/1 -> Add/3
  Delay2/1 -> Gain3/1
  Gain3/1 -> Add/4

== system generic_20231123_1032/CarMaker/VehicleControl/CreateBus VhclCtrl/Stanley steering & speed//Brake controller/Road sensor set & path planning/Road sensor set & path planning/Path_curvature/ Path_expanding ==
  X-path : Inport
  Y_path : Inport  Port=2
  Delay10 : Delay  DelayLength=6
  Delay11 : Delay  DelayLength=8
  Delay37 : Delay
  Delay38 : Delay  DelayLength=4
  Delay4 : Delay
  Delay5 : Delay  DelayLength=6
  Delay6 : Delay  DelayLength=8
  Delay9 : Delay  DelayLength=4
  Mux1 : Mux  Inputs=5
  Mux2 : Mux  Inputs=5
  Reshape1 : Reshape  OutputDimensionality=Customize  OutputDimensions=[1,5]
  Reshape2 : Reshape  OutputDimensionality=Customize  OutputDimensions=[1,5]
  x_path : Outport
  y_path : Outport  Port=2
  wires:
  X-path/1 -> Mux2/1, Delay38/1, Delay37/1, Delay5/1, Delay6/1
  Y_path/1 -> Mux1/1, Delay4/1, Delay9/1, Delay10/1, Delay11/1
  Delay5/1 -> Mux2/4
  Delay37/1 -> Mux2/2
  Delay6/1 -> Mux2/5
  Delay38/1 -> Mux2/3
  Mux1/1 -> Reshape1/1
  Reshape1/1 -> y_path/1
  Delay4/1 -> Mux1/2
  Delay9/1 -> Mux1/3
  Delay10/1 -> Mux1/4
  Delay11/1 -> Mux1/5
  Reshape2/1 -> x_path/1
  Mux2/1 -> Reshape2/1

== system generic_20231123_1032/CarMaker/VehicleControl/CreateBus VhclCtrl/Stanley steering & speed//Brake controller/Road sensor set & path planning/Road sensor set & path planning/Spline_path_planning/Signal_smoothing ==
  Signal_In : Inport
  Smoothing1 : Subsystem
  Smoothing2 : Subsystem
  Smoothing4 : Subsystem
  smoothed_width : Outport
  wires:
  Signal_In/1 -> Smoothing1/1(Signal_In)
  Smoothing1/1(Signal_Out) -> Smoothing2/1(Signal_In)  "steering_signal"
  Smoothing2/1(Signal_Out) -> Smoothing4/1(Signal_In)  "steering_signal"
  Smoothing4/1(Signal_Out) -> smoothed_width/1  "smoothed_width"

== system generic_20231123_1032/CarMaker/VehicleControl/CreateBus VhclCtrl/Stanley steering & speed//Brake controller/Road sensor set & path planning/Road sensor set & path planning/Spline_path_planning/Smoothing3 ==
  Signal_In : Inport
  Add : Sum  Inputs=++++
  Delay : Delay  InitialCondition=0.1
  Delay1 : Delay  DelayLength=4  InitialCondition=0.1
  Delay2 : Delay  DelayLength=5  InitialCondition=0.1
  Gain : Gain  Gain=0.35
  Gain1 : Gain  Gain=0.25
  Gain2 : Gain  Gain=0.25
  Gain3 : Gain  Gain=0.15
  Signal_Out : Outport  VectorParamsAs1DForOutWhenUnconnected=off
  wires:
  Gain3/1 -> Add/4
  Delay2/1 -> Gain3/1
  Gain2/1 -> Add/3
  Add/1 -> Signal_Out/1, Delay/1, Delay1/1, Delay2/1
  Delay1/1 -> Gain2/1
  Gain/1 -> Add/1
  Delay/1 -> Gain1/1
  Signal_In/1 -> Gain/1
  Gain1/1 -> Add/2

== system generic_20231123_1032/CarMaker/VehicleControl/CreateBus VhclCtrl/Stanley steering & speed//Brake controller/Road sensor set & path planning/Road sensor set & path planning/path_planning/Signal_smoothing ==
  Signal_In : Inport
  Smoothing1 : Subsystem
  Smoothing2 : Subsystem
  Smoothing4 : Subsystem
  smoothed_width : Outport
  wires:
  Smoothing4/1(Signal_Out) -> smoothed_width/1  "smoothed_width"
  Smoothing2/1(Signal_Out) -> Smoothing4/1(Signal_In)  "steering_signal"
  Smoothing1/1(Signal_Out) -> Smoothing2/1(Signal_In)  "steering_signal"
  Signal_In/1 -> Smoothing1/1(Signal_In)

== system generic_20231123_1032/CarMaker/VehicleControl/CreateBus VhclCtrl/Stanley steering & speed//Brake controller/Road sensor set & path planning/Road sensor set & path planning/path_planning/Smoothing3 ==
  Signal_In : Inport
  Add : Sum  Inputs=++++
  Delay : Delay  InitialCondition=0.1
  Delay1 : Delay  DelayLength=4  InitialCondition=0.1
  Delay2 : Delay  DelayLength=5  InitialCondition=0.1
  Gain : Gain  Gain=0.35
  Gain1 : Gain  Gain=0.25
  Gain2 : Gain  Gain=0.25
  Gain3 : Gain  Gain=0.15
  Signal_Out : Outport  VectorParamsAs1DForOutWhenUnconnected=off
  wires:
  Gain1/1 -> Add/2
  Signal_In/1 -> Gain/1
  Delay/1 -> Gain1/1
  Gain/1 -> Add/1
  Delay1/1 -> Gain2/1
  Add/1 -> Delay2/1, Delay1/1, Delay/1, Signal_Out/1
  Gain2/1 -> Add/3
  Delay2/1 -> Gain3/1
  Gain3/1 -> Add/4

== system generic_20231123_1032/CarMaker/VehicleControl/CreateBus VhclCtrl/Stanley steering & speed//Brake controller/Stanley_controller_vfin/Stanley_controller_vfin/Stanley_standfort controller/Crosstrack_steering ==
  speed : Inport
  Path.DevDist : Inport  Port=2
  Atan : Trigonometry  Operator=atan
  Divide : Product  Inputs=*/
  Gain : Gain  Gain=-1
  Product : Product
  Sum1 : Sum  Inputs=|++
  k_speed : Constant  Value=k_speed
  k_stanley : Constant  Value=k_stanley
  Cross_track_steering : Outport
  wires:
  Atan/1 -> Cross_track_steering/1
  Divide/1 -> Atan/1
  k_speed/1 -> Sum1/1
  speed/1 -> Sum1/2
  k_stanley/1 -> Product/2
  Sum1/1 -> Divide/2
  Product/1 -> Gain/1
  Gain/1 -> Divide/1
  Path.DevDist/1 -> Product/1

== system generic_20231123_1032/CarMaker/VehicleControl/CreateBus VhclCtrl/Stanley steering & speed//Brake controller/Stanley_controller_vfin/Stanley_controller_vfin/Stanley_standfort controller/Deviation_angle_calc ==
  Velocity : Inport
  Curvature : Inport  Port=2
  Car.YawRate : Inport  Port=3
  Amplifyer : Gain  Gain=Amplifier
  Amplifyer1 : Gain  Gain=10
  Amplifyer2 : Gain  Gain=16.56
  Constant : Constant  Value=2
  Discrete-Time Integrator : DiscreteIntegrator  SampleTime=-1  ICPrevOutput=DiscIntNeverNeededParam  ICPrevScaledInput=DiscIntNeverNeededParam
  Integrator : DiscreteIntegrator  SampleTime=-1  ICPrevOutput=DiscIntNeverNeededParam  ICPrevScaledInput=DiscIntNeverNeededParam
  Multiport Switch : MultiPortSwitch  Inputs=2  SaturateOnIntegerOverflow=off  InputSameDT=off
  Product : Product
  Read CM Dict : CarMaker4SL/Read CM Dict  xname=Sensor.Road.VehSensor_0.Path.DevAng  xsync=off  xstime=Continuous
  Scope : Scope  NumInputPorts=2
  Sum3 : Sum  Inputs=|+-
  Switch : Switch  Criteria=u2 > Threshold  SaturateOnIntegerOverflow=off  InputSameDT=off
  Dev_angle : Outport
  wires:
  Amplifyer1/1 -> Switch/3  "Dev_angle"
  Curvature/1 -> Product/1
  Car.YawRate/1 -> Discrete-Time Integrator/1
  Velocity/1 -> Product/2
  Product/1 -> Integrator/1
  Integrator/1 -> Sum3/1  "Dev_angle"
  Discrete-Time Integrator/1 -> Sum3/2
  Amplifyer2/1 -> Switch/1  "Dev_angle"
  Sum3/1 -> Amplifyer1/1, Switch/2, Amplifyer2/1  "heading_error"
  Switch/1 -> Scope/1, Multiport Switch/2  "Dev_angle"
  Amplifyer/1 -> Scope/2, Multiport Switch/3  "Dev_angle"
  Read CM Dict/1 -> Amplifyer/1
  Constant/1 -> Multiport Switch/1
  Multiport Switch/1 -> Dev_angle/1  "Dev_angle"

== system generic_20231123_1032/CarMaker/VehicleControl/CreateBus VhclCtrl/Stanley steering & speed//Brake controller/Stanley_controller_vfin/Stanley_controller_vfin/Stanley_standfort controller/Steady_state_yaw ==
  V : Inport
  Curvature : Inport  Port=2
  Car_Yaw_rate : Inport  Port=3
  Discrete-Time Integrator : DiscreteIntegrator  SampleTime=-1  ICPrevOutput=DiscIntNeverNeededParam  ICPrevScaledInput=DiscIntNeverNeededParam
  Steady_state_yaw : Subsystem
  Sum : Sum  Inputs=|-+
  Steady_state_yaw1 : Outport
  wires:
  V/1 -> Steady_state_yaw/1(V)
  Sum/1 -> Steady_state_yaw1/1  "Steady_state_yaw"
  Steady_state_yaw/1(Steady_state_yaw) -> Sum/1  "Steady_state_yaw"
  Discrete-Time Integrator/1 -> Sum/2
  Car_Yaw_rate/1 -> Discrete-Time Integrator/1
  Curvature/1 -> Steady_state_yaw/2(Curvature)

== system generic_20231123_1032/CarMaker/VehicleControl/CreateBus VhclCtrl/Stanley steering & speed//Brake controller/Stanley_controller_vfin/Stanley_controller_vfin/Stanley_standfort controller/Steering_correction_facotr ==
  Steering_i+1 : Inport
  Steering_i : Inport  Port=2
  K_dsteering : Constant  Value=K_dsteering
  Memory : Memory  LinearizeAsDelay=on
  Product2 : Product
  Sum2 : Sum  Inputs=|+-
  Factor_of_correction : Outport
  wires:
  K_dsteering/1 -> Product2/1
  Memory/1 -> Sum2/1
  Sum2/1 -> Product2/2
  Steering_i+1/1 -> Sum2/2
  Steering_i/1 -> Memory/1
  Product2/1 -> Factor_of_correction/1

== system generic_20231123_1032/CarMaker/VehicleControl/CreateBus VhclCtrl/Stanley steering & speed//Brake controller/Stanley_controller_vfin/Stanley_controller_vfin/Stanley_standfort controller/Yaw_rate_diff ==
  Velocity : Inport
  Curvature : Inport  Port=2
  Car_yaw_rate : Inport  Port=3
  K_d_yawrate : Constant  Value=K_d_yawrate
  Product : Product
  Product1 : Product
  Sum1 : Sum  Inputs=|+-
  Yaw_rate_factor : Outport
  wires:
  K_d_yawrate/1 -> Product1/1
  Car_yaw_rate/1 -> Sum1/2
  Velocity/1 -> Product/1
  Curvature/1 -> Product/2
  Sum1/1 -> Product1/2
  Product/1 -> Sum1/1
  Product1/1 -> Yaw_rate_factor/1

== system generic_20231123_1032/CarMaker/VehicleControl/CreateBus VhclCtrl/Stanley steering & speed//Brake controller/Road sensor set & path planning/Road sensor set & path planning/A* star path planning/Signal_smoothing/Smoothing1 ==
  Signal_In : Inport
  Add : Sum  Inputs=++++
  Delay : Delay  InitialCondition=0.1
  Delay1 : Delay  DelayLength=4  InitialCondition=0.1
  Delay2 : Delay  DelayLength=5  InitialCondition=0.1
  Gain : Gain  Gain=0.35
  Gain1 : Gain  Gain=0.25
  Gain2 : Gain  Gain=0.25
  Gain3 : Gain  Gain=0.15
  Signal_Out : Outport  VectorParamsAs1DForOutWhenUnconnected=off
  wires:
  Gain1/1 -> Add/2
  Signal_In/1 -> Gain/1
  Delay/1 -> Gain1/1
  Gain/1 -> Add/1
  Delay1/1 -> Gain2/1
  Add/1 -> Delay2/1, Delay1/1, Delay/1, Signal_Out/1
  Gain2/1 -> Add/3
  Delay2/1 -> Gain3/1
  Gain3/1 -> Add/4

== system generic_20231123_1032/CarMaker/VehicleControl/CreateBus VhclCtrl/Stanley steering & speed//Brake controller/Road sensor set & path planning/Road sensor set & path planning/A* star path planning/Signal_smoothing/Smoothing2 ==
  Signal_In : Inport
  Add : Sum  Inputs=++++
  Delay : Delay  InitialCondition=0.1
  Delay1 : Delay  DelayLength=4  InitialCondition=0.1
  Delay2 : Delay  DelayLength=5  InitialCondition=0.1
  Gain : Gain  Gain=0.35
  Gain1 : Gain  Gain=0.25
  Gain2 : Gain  Gain=0.25
  Gain3 : Gain  Gain=0.15
  Signal_Out : Outport  VectorParamsAs1DForOutWhenUnconnected=off
  wires:
  Gain3/1 -> Add/4
  Delay2/1 -> Gain3/1
  Gain2/1 -> Add/3
  Add/1 -> Signal_Out/1, Delay/1, Delay1/1, Delay2/1
  Delay1/1 -> Gain2/1
  Gain/1 -> Add/1
  Delay/1 -> Gain1/1
  Signal_In/1 -> Gain/1
  Gain1/1 -> Add/2

== system generic_20231123_1032/CarMaker/VehicleControl/CreateBus VhclCtrl/Stanley steering & speed//Brake controller/Road sensor set & path planning/Road sensor set & path planning/A* star path planning/Signal_smoothing/Smoothing4 ==
  Signal_In : Inport
  Add : Sum  Inputs=++++
  Delay : Delay  InitialCondition=0.1
  Delay1 : Delay  DelayLength=4  InitialCondition=0.1
  Delay2 : Delay  DelayLength=5  InitialCondition=0.1
  Gain : Gain  Gain=0.35
  Gain1 : Gain  Gain=0.25
  Gain2 : Gain  Gain=0.25
  Gain3 : Gain  Gain=0.15
  Signal_Out : Outport  VectorParamsAs1DForOutWhenUnconnected=off
  wires:
  Gain1/1 -> Add/2
  Signal_In/1 -> Gain/1
  Delay/1 -> Gain1/1
  Gain/1 -> Add/1
  Delay1/1 -> Gain2/1
  Add/1 -> Delay2/1, Delay1/1, Delay/1, Signal_Out/1
  Gain2/1 -> Add/3
  Delay2/1 -> Gain3/1
  Gain3/1 -> Add/4

== system generic_20231123_1032/CarMaker/VehicleControl/CreateBus VhclCtrl/Stanley steering & speed//Brake controller/Road sensor set & path planning/Road sensor set & path planning/Be'zeir path planning/Signal_smoothing/Smoothing1 ==
  Signal_In : Inport
  Add : Sum  Inputs=++++
  Delay : Delay  InitialCondition=0.1
  Delay1 : Delay  DelayLength=4  InitialCondition=0.1
  Delay2 : Delay  DelayLength=5  InitialCondition=0.1
  Gain : Gain  Gain=0.35
  Gain1 : Gain  Gain=0.25
  Gain2 : Gain  Gain=0.25
  Gain3 : Gain  Gain=0.15
  Signal_Out : Outport  VectorParamsAs1DForOutWhenUnconnected=off
  wires:
  Gain3/1 -> Add/4
  Delay2/1 -> Gain3/1
  Gain2/1 -> Add/3
  Add/1 -> Signal_Out/1, Delay/1, Delay1/1, Delay2/1
  Delay1/1 -> Gain2/1
  Gain/1 -> Add/1
  Delay/1 -> Gain1/1
  Signal_In/1 -> Gain/1
  Gain1/1 -> Add/2

== system generic_20231123_1032/CarMaker/VehicleControl/CreateBus VhclCtrl/Stanley steering & speed//Brake controller/Road sensor set & path planning/Road sensor set & path planning/Be'zeir path planning/Signal_smoothing/Smoothing2 ==
  Signal_In : Inport
  Add : Sum  Inputs=++++
  Delay : Delay  InitialCondition=0.1
  Delay1 : Delay  DelayLength=4  InitialCondition=0.1
  Delay2 : Delay  DelayLength=5  InitialCondition=0.1
  Gain : Gain  Gain=0.35
  Gain1 : Gain  Gain=0.25
  Gain2 : Gain  Gain=0.25
  Gain3 : Gain  Gain=0.15
  Signal_Out : Outport  VectorParamsAs1DForOutWhenUnconnected=off
  wires:
  Gain1/1 -> Add/2
  Signal_In/1 -> Gain/1
  Delay/1 -> Gain1/1
  Gain/1 -> Add/1
  Delay1/1 -> Gain2/1
  Add/1 -> Delay2/1, Delay1/1, Delay/1, Signal_Out/1
  Gain2/1 -> Add/3
  Delay2/1 -> Gain3/1
  Gain3/1 -> Add/4

== system generic_20231123_1032/CarMaker/VehicleControl/CreateBus VhclCtrl/Stanley steering & speed//Brake controller/Road sensor set & path planning/Road sensor set & path planning/Be'zeir path planning/Signal_smoothing/Smoothing4 ==
  Signal_In : Inport
  Add : Sum  Inputs=++++
  Delay : Delay  InitialCondition=0.1
  Delay1 : Delay  DelayLength=4  InitialCondition=0.1
  Delay2 : Delay  DelayLength=5  InitialCondition=0.1
  Gain : Gain  Gain=0.35
  Gain1 : Gain  Gain=0.25
  Gain2 : Gain  Gain=0.25
  Gain3 : Gain  Gain=0.15
  Signal_Out : Outport  VectorParamsAs1DForOutWhenUnconnected=off
  wires:
  Gain3/1 -> Add/4
  Delay2/1 -> Gain3/1
  Gain2/1 -> Add/3
  Add/1 -> Signal_Out/1, Delay/1, Delay1/1, Delay2/1
  Delay1/1 -> Gain2/1
  Gain/1 -> Add/1
  Delay/1 -> Gain1/1
  Signal_In/1 -> Gain/1
  Gain1/1 -> Add/2

== system generic_20231123_1032/CarMaker/VehicleControl/CreateBus VhclCtrl/Stanley steering & speed//Brake controller/Road sensor set & path planning/Road sensor set & path planning/Dijkestra path planning/Signal_smoothing/Smoothing1 ==
  Signal_In : Inport
  Add : Sum  Inputs=++++
  Delay : Delay  InitialCondition=0.1
  Delay1 : Delay  DelayLength=4  InitialCondition=0.1
  Delay2 : Delay  DelayLength=5  InitialCondition=0.1
  Gain : Gain  Gain=0.35
  Gain1 : Gain  Gain=0.25
  Gain2 : Gain  Gain=0.25
  Gain3 : Gain  Gain=0.15
  Signal_Out : Outport  VectorParamsAs1DForOutWhenUnconnected=off
  wires:
  Gain3/1 -> Add/4
  Delay2/1 -> Gain3/1
  Gain2/1 -> Add/3
  Add/1 -> Signal_Out/1, Delay/1, Delay1/1, Delay2/1
  Delay1/1 -> Gain2/1
  Gain/1 -> Add/1
  Delay/1 -> Gain1/1
  Signal_In/1 -> Gain/1
  Gain1/1 -> Add/2

== system generic_20231123_1032/CarMaker/VehicleControl/CreateBus VhclCtrl/Stanley steering & speed//Brake controller/Road sensor set & path planning/Road sensor set & path planning/Dijkestra path planning/Signal_smoothing/Smoothing2 ==
  Signal_In : Inport
  Add : Sum  Inputs=++++
  Delay : Delay  InitialCondition=0.1
  Delay1 : Delay  DelayLength=4  InitialCondition=0.1
  Delay2 : Delay  DelayLength=5  InitialCondition=0.1
  Gain : Gain  Gain=0.35
  Gain1 : Gain  Gain=0.25
  Gain2 : Gain  Gain=0.25
  Gain3 : Gain  Gain=0.15
  Signal_Out : Outport  VectorParamsAs1DForOutWhenUnconnected=off
  wires:
  Gain1/1 -> Add/2
  Signal_In/1 -> Gain/1
  Delay/1 -> Gain1/1
  Gain/1 -> Add/1
  Delay1/1 -> Gain2/1
  Add/1 -> Delay2/1, Delay1/1, Delay/1, Signal_Out/1
  Gain2/1 -> Add/3
  Delay2/1 -> Gain3/1
  Gain3/1 -> Add/4
